simulink subsystem "Actuators"  (R2020a)
settings: Solver=VariableStepAuto  StartTime=0.0  StopTime=10.0  RelTol=1e-3
settings Model: Creator=decla  LastModifiedBy=decla

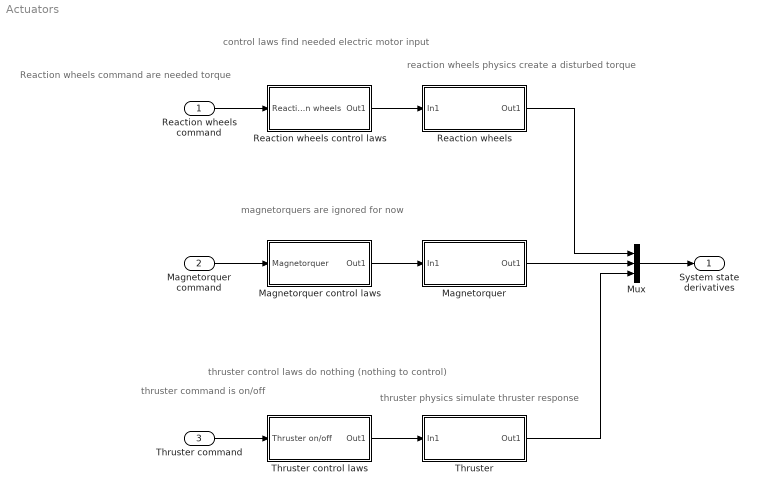
== system Actuators ==
  note: magnetorquers are ignored for now
  note: thruster control laws do nothing (nothing to control)
  note: thruster physics simulate thruster response
  note: thruster command is on/off
  note: reaction wheels physics create a disturbed torque
  note: control laws find needed electric motor input
  note: Reaction wheels command are needed torque
  Reaction wheels command : Inport
  Magnetorquer command : Inport  Port=2
  Thruster command : Inport  Port=3
  Magnetorquer : Subsystem
  Magnetorquer control laws : Subsystem
  Mux : Mux  Inputs=3
  Reaction wheels : Subsystem
  Reaction wheels control laws : Subsystem
  Thruster : Subsystem
  Thruster control laws : Subsystem
  System state derivatives : Outport
  wires:
  Reaction wheels command/1 -> Reaction wheels control laws/1(Reaction wheels)
  Magnetorquer command/1 -> Magnetorquer control laws/1(Magnetorquer)
  Thruster command/1 -> Thruster control laws/1(Thruster on/off)
  Thruster control laws/1(Out1) -> Thruster/1(In1)
  Magnetorquer control laws/1(Out1) -> Magnetorquer/1(In1)
  Reaction wheels control laws/1(Out1) -> Reaction wheels/1(In1)
  Thruster/1(Out1) -> Mux/3
  Magnetorquer/1(Out1) -> Mux/2
  Reaction wheels/1(Out1) -> Mux/1
  Mux/1 -> System state derivatives/1

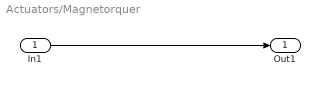
== system Actuators/Magnetorquer ==
  In1 : Inport
  Out1 : Outport
  wires:
  In1/1 -> Out1/1

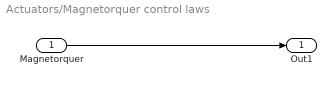
== system Actuators/Magnetorquer control laws ==
  Magnetorquer : Inport
  Out1 : Outport
  wires:
  Magnetorquer/1 -> Out1/1

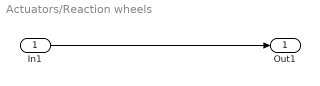
== system Actuators/Reaction wheels ==
  In1 : Inport
  Out1 : Outport
  wires:
  In1/1 -> Out1/1

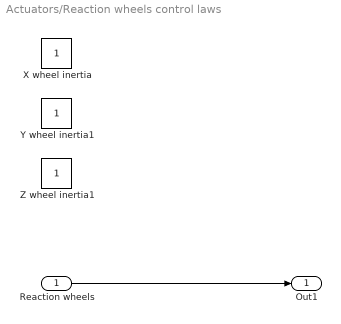
== system Actuators/Reaction wheels control laws ==
  Reaction wheels : Inport
  X wheel inertia : Constant
  Y wheel inertia1 : Constant
  Z wheel inertia1 : Constant
  Out1 : Outport
  wires:
  Reaction wheels/1 -> Out1/1

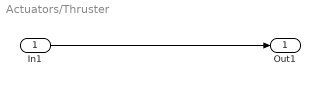
== system Actuators/Thruster ==
  In1 : Inport
  Out1 : Outport
  wires:
  In1/1 -> Out1/1

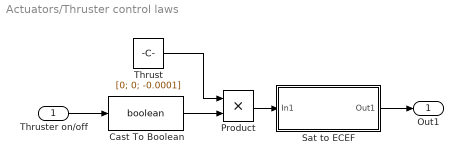
== system Actuators/Thruster control laws ==
  Thruster on/off : Inport
  Cast To Boolean : DataTypeConversion  OutDataTypeStr=boolean
  Product : Product
  Sat to ECEF : Subsystem
  Thrust : Constant  Value=[0; 0; -0.0001]
  Out1 : Outport
  wires:
  Sat to ECEF/1(Out1) -> Out1/1
  Product/1 -> Sat to ECEF/1(In1)
  Thrust/1 -> Product/1
  Cast To Boolean/1 -> Product/2
  Thruster on/off/1 -> Cast To Boolean/1

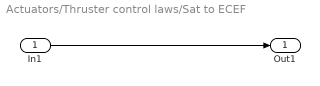
== system Actuators/Thruster control laws/Sat to ECEF ==
  In1 : Inport
  Out1 : Outport
  wires:
  In1/1 -> Out1/1
